simulink model "test_rapidaccel_sfunc_nrlmsise00_2"  (Simulink 7.8)
settings: Solver=ode4  StartTime=0.0  StopTime=100000  FixedStep=0.1  RelTol=1e-3
settings Model: Creator=kkamiya  LastModifiedBy=kkamiya  SimulationMode=rapid-accelerator
settings SFSimCC: SimUserSources=|
  | sfunc_nrlmsise00_wrapper.c
  | nrlmsise-00.c
  | nrlmsise-00_data.c

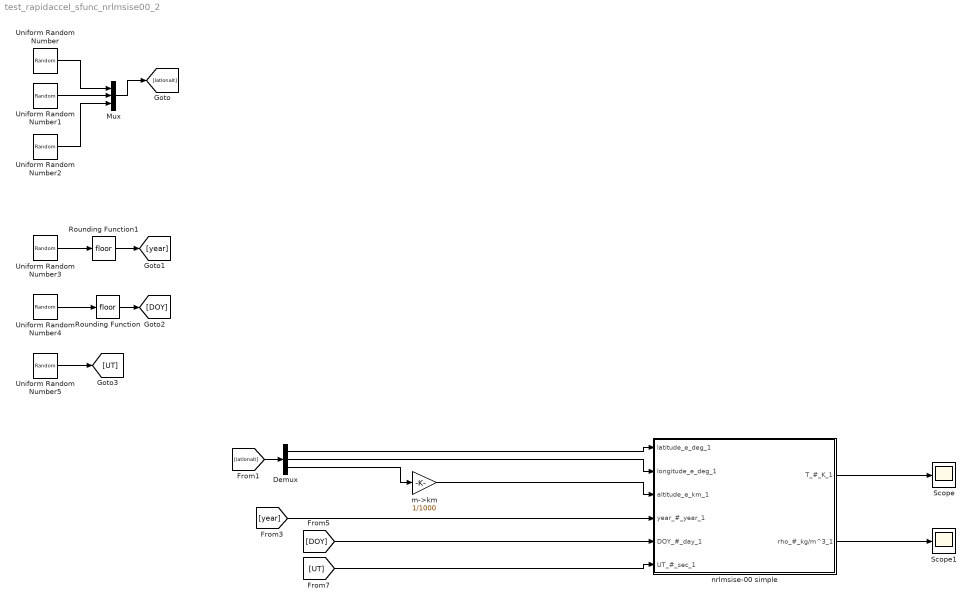
== system test_rapidaccel_sfunc_nrlmsise00_2 ==
  Demux : Demux  Outputs=3
  Mux : Mux  Inputs=3
  Rounding Function : Rounding
  Rounding Function1 : Rounding
  Scope : Scope
      settings: YMin=750  YMax=1350
  Scope1 : Scope
      settings: YMin=8.07794e-028  YMax=3e-011
  Uniform Random Number : UniformRandomNumber  Minimum=-90  Maximum=90  Seed=-1  SampleTime=0.1
  Uniform Random Number1 : UniformRandomNumber  Minimum=0  Maximum=360  Seed=-2  SampleTime=0.1
  Uniform Random Number2 : UniformRandomNumber  Minimum=300000  Maximum=800000  Seed=-3  SampleTime=0.1
  Uniform Random Number3 : UniformRandomNumber  Minimum=1950  Maximum=2050  Seed=-4  SampleTime=0.1
  Uniform Random Number4 : UniformRandomNumber  Minimum=0  Maximum=365  Seed=-5  SampleTime=0.1
  Uniform Random Number5 : UniformRandomNumber  Minimum=0  Maximum=86400  Seed=-6  SampleTime=0.1
  m->km : Gain  Gain=1/1000
  nrlmsise-00 simple : Subsystem
  wires:
  Uniform Random Number3/1 -> Rounding Function1/1
  Uniform Random Number5/1 -> [UT]
  [latlonalt] -> Demux/1
  Demux/1 -> nrlmsise-00 simple/1(latitude_e_deg_1)
  Demux/3 -> m->km/1
  [year] -> nrlmsise-00 simple/4(year_#_year_1)
  [DOY] -> nrlmsise-00 simple/5(DOY_#_day_1)
  m->km/1 -> nrlmsise-00 simple/3(altitude_e_km_1)
  Uniform Random Number/1 -> Mux/1
  Uniform Random Number1/1 -> Mux/2
  Mux/1 -> [latlonalt]
  Uniform Random Number2/1 -> Mux/3
  Uniform Random Number4/1 -> Rounding Function/1
  Rounding Function/1 -> [DOY]
  Demux/2 -> nrlmsise-00 simple/2(longitude_e_deg_1)
  [UT] -> nrlmsise-00 simple/6(UT_#_sec_1)
  Rounding Function1/1 -> [year]
  nrlmsise-00 simple/1(T_#_K_1) -> Scope/1
  nrlmsise-00 simple/2(rho_#_kg/m^3_1) -> Scope1/1

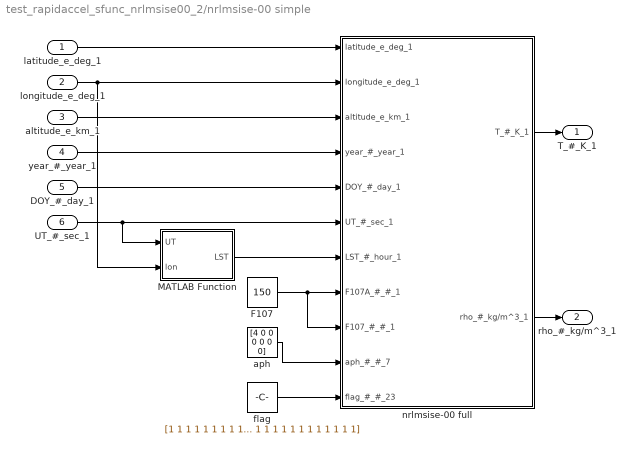
== system test_rapidaccel_sfunc_nrlmsise00_2/nrlmsise-00 simple ==
  latitude_e_deg_1 : Inport
  longitude_e_deg_1 : Inport  Port=2
  altitude_e_km_1 : Inport  Port=3
  year_#_year_1 : Inport  Port=4
  DOY_#_day_1 : Inport  Port=5
  UT_#_sec_1 : Inport  Port=6
  F107 : Constant  Value=150
  MATLAB Function : MATLAB Function  TreatAsAtomicUnit=on
  aph : Constant  Value=[4 0 0 0 0 0 0]
  flag : Constant  Value=[1 1 1 1 1 1 1 1 1 1 1 1 1 1 1 1 1 1 1 1 1 1 1]
  nrlmsise-00 full : Subsystem
  T_#_K_1 : Outport
  rho_#_kg/m^3_1 : Outport  Port=2
  wires:
  longitude_e_deg_1/1 -> MATLAB Function/2(lon), nrlmsise-00 full/2(longitude_e_deg_1)
  UT_#_sec_1/1 -> MATLAB Function/1(UT), nrlmsise-00 full/6(UT_#_sec_1)
  flag/1 -> nrlmsise-00 full/11(flag_#_#_23)
  aph/1 -> nrlmsise-00 full/10(aph_#_#_7)
  F107/1 -> nrlmsise-00 full/8(F107A_#_#_1), nrlmsise-00 full/9(F107_#_#_1)
  MATLAB Function/1(LST) -> nrlmsise-00 full/7(LST_#_hour_1)
  latitude_e_deg_1/1 -> nrlmsise-00 full/1(latitude_e_deg_1)
  altitude_e_km_1/1 -> nrlmsise-00 full/3(altitude_e_km_1)
  nrlmsise-00 full/1(T_#_K_1) -> T_#_K_1/1
  year_#_year_1/1 -> nrlmsise-00 full/4(year_#_year_1)
  DOY_#_day_1/1 -> nrlmsise-00 full/5(DOY_#_day_1)
  nrlmsise-00 full/2(rho_#_kg/m^3_1) -> rho_#_kg/m^3_1/1

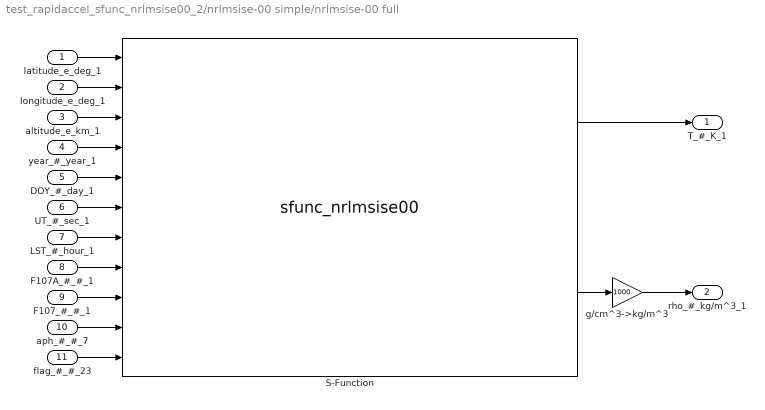
== system test_rapidaccel_sfunc_nrlmsise00_2/nrlmsise-00 simple/nrlmsise-00 full ==
  latitude_e_deg_1 : Inport
  longitude_e_deg_1 : Inport  Port=2
  altitude_e_km_1 : Inport  Port=3
  year_#_year_1 : Inport  Port=4
  DOY_#_day_1 : Inport  Port=5
  UT_#_sec_1 : Inport  Port=6
  LST_#_hour_1 : Inport  Port=7
  F107A_#_#_1 : Inport  Port=8
  F107_#_#_1 : Inport  Port=9
  aph_#_#_7 : Inport  Port=10
  flag_#_#_23 : Inport  Port=11
  S-Function : S-Function  FunctionName=sfunc_nrlmsise00  EnableBusSupport=off
  g/cm^3->kg/m^3 : Gain  Gain=1000
  T_#_K_1 : Outport
  rho_#_kg/m^3_1 : Outport  Port=2
  wires:
  S-Function/2 -> g/cm^3->kg/m^3/1
  latitude_e_deg_1/1 -> S-Function/1
  longitude_e_deg_1/1 -> S-Function/2
  altitude_e_km_1/1 -> S-Function/3
  S-Function/1 -> T_#_K_1/1
  year_#_year_1/1 -> S-Function/4
  DOY_#_day_1/1 -> S-Function/5
  UT_#_sec_1/1 -> S-Function/6
  LST_#_hour_1/1 -> S-Function/7
  F107A_#_#_1/1 -> S-Function/8
  g/cm^3->kg/m^3/1 -> rho_#_kg/m^3_1/1
  F107_#_#_1/1 -> S-Function/9
  aph_#_#_7/1 -> S-Function/10
  flag_#_#_23/1 -> S-Function/11

== matlab function nrlmsise-00 simple/MATLAB Function ==
  data: UT input double; LST output double; lon input double
function LST = fcn(UT,lon)
%#codegen

LST = UT / 3600 + lon / 15;
